simulink model "CL"  (R2017b)
settings: Solver=VariableStepAuto  StartTime=0.0  StopTime=10.0  RelTol=1e-3
values from neighbouring files (symbols this model uses):
  CL0 = 0.307    [Cessna_Simulation.m]
  CLa = 4.41    [Cessna_Simulation.m]
  CLadot = 1.7    [Cessna_Simulation.m]
  CLel = 0.43    [Cessna_Simulation.m]
  CLq = 3.9    [Cessna_Simulation.m]
undefined symbols (not defined in the file or in its folder): cbar
settings Model: Creator=stroll  LastModifiedBy=stroll

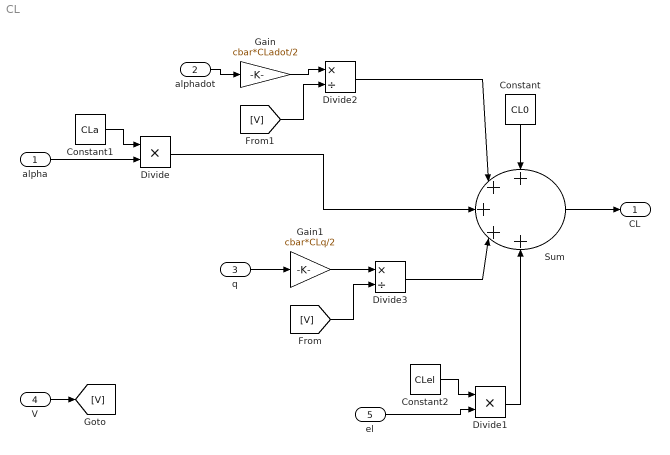
== system CL ==
  alpha : Inport
  alphadot : Inport  Port=2
  q : Inport  Port=3
  V : Inport  Port=4
  el : Inport  Port=5
  Constant : Constant  Value=CL0
  Constant1 : Constant  Value=CLa
  Constant2 : Constant  Value=CLel
  Divide : Product
  Divide1 : Product
  Divide2 : Product  Inputs=*/
  Divide3 : Product  Inputs=*/
  Gain : Gain  Gain=cbar*CLadot/2
  Gain1 : Gain  Gain=cbar*CLq/2
  Sum : Sum  Inputs=+++++
  CL : Outport
  wires:
  Sum/1 -> CL/1
  Constant/1 -> Sum/1
  Constant1/1 -> Divide/1
  alpha/1 -> Divide/2
  alphadot/1 -> Gain/1
  Gain/1 -> Divide2/1
  Gain1/1 -> Divide3/1
  q/1 -> Gain1/1
  V/1 -> [V]
  [V] -> Divide3/2
  [V] -> Divide2/2
  Divide2/1 -> Sum/2
  Divide/1 -> Sum/3
  Divide3/1 -> Sum/4
  el/1 -> Divide1/2
  Constant2/1 -> Divide1/1
  Divide1/1 -> Sum/5
